simulink model "SDT505SimpleMotorModelPowerOutput220119"  (R2022b)
settings: Solver=VariableStepAuto  StartTime=0.0  StopTime=10.0  RelTol=1e-3
undefined symbols (not defined in the file or in its folder): m
libraries: simulink x4
settings Model: Creator=mjbou  LastModifiedBy=mjbou
settings SolverCC: AlgebraicLoopSolver=TrustRegion
settings DebuggingCC: UnconnectedInputMsg=warning  UnconnectedOutputMsg=warning  UnconnectedLineMsg=warning  SFMachineParentedDataDiag=warning
settings ModelReferenceCC: EnableRefExpFcnMdlSchedulingChecks=on

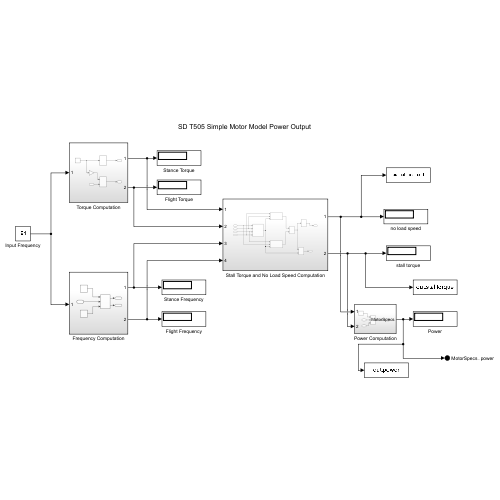
[thumbnail: Simulink's stored preview of the top-level diagram]
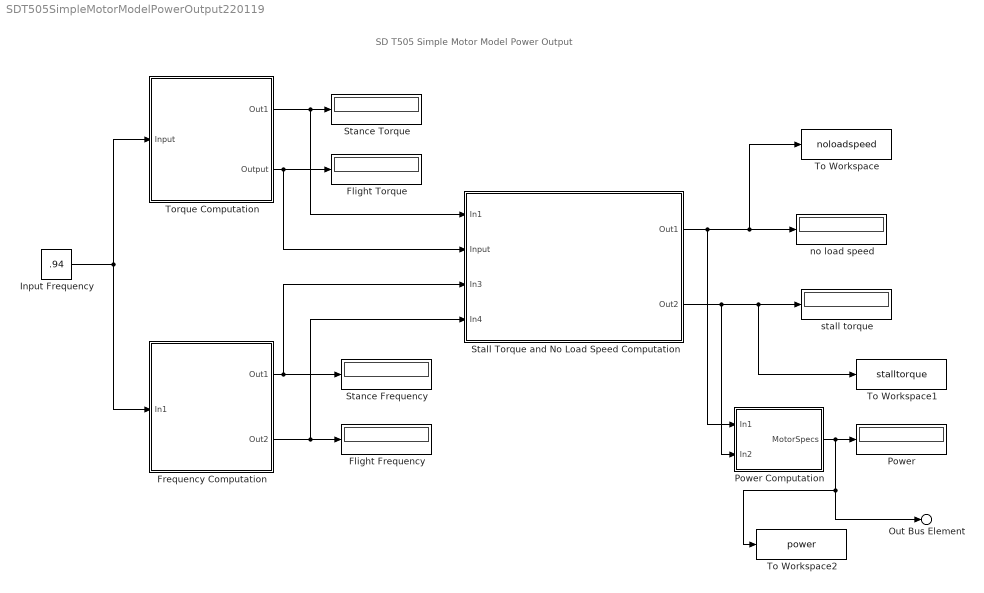
== system SDT505SimpleMotorModelPowerOutput220119 ==
  note: SD T505 Simple Motor Model Power Output
  Flight Frequency : Display
  Flight Torque : Display
  Frequency Computation : Subsystem
  Input Frequency : Constant  Value=.94
  Power : Display
  Power Computation : Subsystem
  Stall Torque and No Load Speed Computation : Subsystem
  Stance Frequency : Display
  Stance Torque : Display
  To Workspace : ToWorkspace  VariableName=noloadspeed  SaveFormat=Timeseries  SampleTime=-1
  To Workspace1 : ToWorkspace  VariableName=stalltorque  SaveFormat=Timeseries  SampleTime=-1
  To Workspace2 : ToWorkspace  VariableName=power  SaveFormat=Timeseries  SampleTime=-1
  Torque Computation : Subsystem
  no load speed : Display
  stall torque : Display
  Out Bus Element : Outport  PortName=MotorSpecs  Element=power
  wires:
  Frequency Computation/2(Out2) -> Stall Torque and No Load Speed Computation/4(In4), Flight Frequency/1
  Input Frequency/1 -> Torque Computation/1(Input), Frequency Computation/1(In1)
  Torque Computation/1(Out1) -> Stance Torque/1, Stall Torque and No Load Speed Computation/1(In1)
  Torque Computation/2(Output) -> Flight Torque/1, Stall Torque and No Load Speed Computation/2(Input)
  Stall Torque and No Load Speed Computation/1(Out1) -> Power Computation/1(In1), To Workspace/1, no load speed/1
  Stall Torque and No Load Speed Computation/2(Out2) -> Power Computation/2(In2), To Workspace1/1, stall torque/1
  Frequency Computation/1(Out1) -> Stance Frequency/1, Stall Torque and No Load Speed Computation/3(In3)
  Power Computation/1(MotorSpecs) -> To Workspace2/1, Out Bus Element/1, Power/1

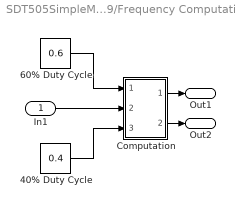
== system SDT505SimpleMotorModelPowerOutput220119/Frequency Computation ==
  In1 : Inport
  40% Duty Cycle : Constant  Value=0.4
  60% Duty Cycle : Constant  Value=0.6
  Computation : Subsystem
  Out1 : Outport
  Out2 : Outport  Port=2
  wires:
  60% Duty Cycle/1 -> Computation/1(In1)
  In1/1 -> Computation/2(In2)
  40% Duty Cycle/1 -> Computation/3(In3)
  Computation/1(Out1) -> Out1/1
  Computation/2(Out2) -> Out2/1

== system SDT505SimpleMotorModelPowerOutput220119/Power Computation ==
  In1 : Inport
  In2 : Inport  Port=2
  Constant : Constant  Value=0.25
  Product : Product  Inputs=3
  MotorSpecs : Outport
  wires:
  Constant/1 -> Product/1
  In2/1 -> Product/3
  In1/1 -> Product/2
  Product/1 -> MotorSpecs/1

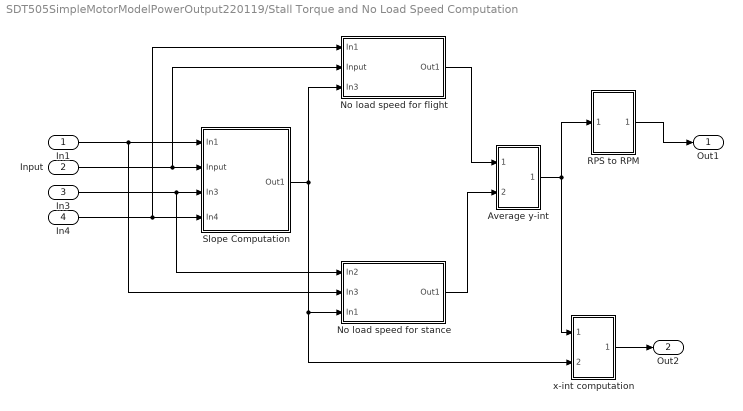
== system SDT505SimpleMotorModelPowerOutput220119/Stall Torque and No Load Speed Computation ==
  In1 : Inport
  Input : Inport  Port=2
  In3 : Inport  Port=3
  In4 : Inport  Port=4
  Average y-int : Subsystem
  No load speed for flight : Subsystem
  No load speed for stance : Subsystem
  RPS to RPM : Subsystem
  Slope Computation : Subsystem
  x-int computation : Subsystem
  Out1 : Outport
  Out2 : Outport  Port=2
  wires:
  No load speed for flight/1(Out1) -> Average y-int/1(In1)
  No load speed for stance/1(Out1) -> Average y-int/2(In2)
  Slope Computation/1(Out1) -> No load speed for flight/3(In3), x-int computation/2(In2), No load speed for stance/3(In1)
  x-int computation/1(Out1) -> Out2/1
  Average y-int/1(Out1) -> x-int computation/1(In1), RPS to RPM/1(In1)
  In3/1 -> No load speed for stance/1(In2), Slope Computation/3(In3)
  In1/1 -> No load speed for stance/2(In3), Slope Computation/1(In1)
  Input/1 -> No load speed for flight/2(Input), Slope Computation/2(Input)
  In4/1 -> No load speed for flight/1(In1), Slope Computation/4(In4)
  RPS to RPM/1(Out1) -> Out1/1

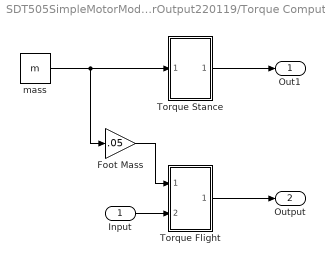
== system SDT505SimpleMotorModelPowerOutput220119/Torque Computation ==
  Input : Inport
  Foot Mass : Gain  Gain=.05
  Torque Flight : Subsystem
  Torque Stance : Subsystem
  mass : Constant  Value=m
  Out1 : Outport
  Output : Outport  Port=2
  wires:
  Torque Flight/1(Out2) -> Output/1
  Input/1 -> Torque Flight/2(Input)
  Torque Stance/1(Out1) -> Out1/1
  Foot Mass/1 -> Torque Flight/1(In1)
  mass/1 -> Foot Mass/1, Torque Stance/1(In1)

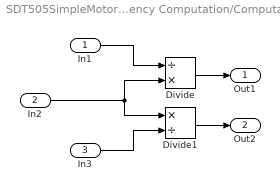
== system SDT505SimpleMotorModelPowerOutput220119/Frequency Computation/Computation ==
  In1 : Inport
  In2 : Inport  Port=2
  In3 : Inport  Port=3
  Divide : Product  Inputs=/*
  Divide1 : Product  Inputs=*/
  Out1 : Outport
  Out2 : Outport  Port=2
  wires:
  In2/1 -> Divide1/1, Divide/2
  Divide/1 -> Out1/1
  In3/1 -> Divide1/2
  In1/1 -> Divide/1
  Divide1/1 -> Out2/1

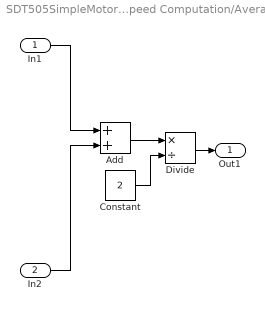
== system SDT505SimpleMotorModelPowerOutput220119/Stall Torque and No Load Speed Computation/Average y-int ==
  In1 : Inport
  In2 : Inport  Port=2
  Add : Sum
  Constant : Constant  Value=2
  Divide : Product  Inputs=*/
  Out1 : Outport
  wires:
  Divide/1 -> Out1/1
  Constant/1 -> Divide/2
  Add/1 -> Divide/1
  In1/1 -> Add/1
  In2/1 -> Add/2

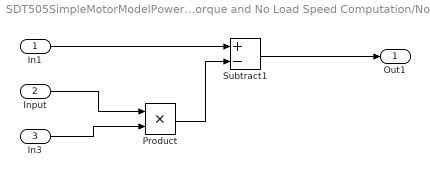
== system SDT505SimpleMotorModelPowerOutput220119/Stall Torque and No Load Speed Computation/No load speed for flight ==
  In1 : Inport
  Input : Inport  Port=2
  In3 : Inport  Port=3
  Product : Product
  Subtract1 : Sum  Inputs=+-
  Out1 : Outport
  wires:
  Input/1 -> Product/1
  In3/1 -> Product/2
  In1/1 -> Subtract1/1
  Product/1 -> Subtract1/2
  Subtract1/1 -> Out1/1

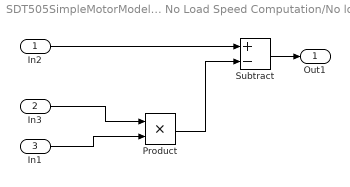
== system SDT505SimpleMotorModelPowerOutput220119/Stall Torque and No Load Speed Computation/No load speed for stance ==
  In2 : Inport
  In3 : Inport  Port=2
  In1 : Inport  Port=3
  Product : Product
  Subtract : Sum  Inputs=+-
  Out1 : Outport
  wires:
  Subtract/1 -> Out1/1
  Product/1 -> Subtract/2
  In3/1 -> Product/1
  In1/1 -> Product/2
  In2/1 -> Subtract/1

== system SDT505SimpleMotorModelPowerOutput220119/Stall Torque and No Load Speed Computation/RPS to RPM ==
  In1 : Inport
  Constant : Constant  Value=60
  Product : Product
  Out1 : Outport
  wires:
  In1/1 -> Product/2
  Product/1 -> Out1/1
  Constant/1 -> Product/1

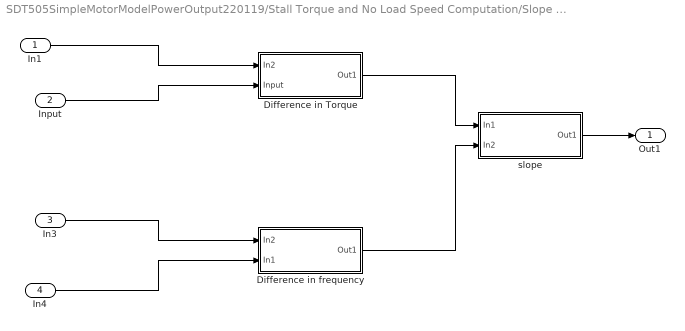
== system SDT505SimpleMotorModelPowerOutput220119/Stall Torque and No Load Speed Computation/Slope Computation ==
  In1 : Inport
  Input : Inport  Port=2
  In3 : Inport  Port=3
  In4 : Inport  Port=4
  Difference in Torque : Subsystem
  Difference in frequency : Subsystem
  slope : Subsystem
  Out1 : Outport
  wires:
  Difference in frequency/1(Out1) -> slope/2(In2)
  Difference in Torque/1(Out1) -> slope/1(In1)
  slope/1(Out1) -> Out1/1
  Input/1 -> Difference in Torque/2(Input)
  In4/1 -> Difference in frequency/2(In1)
  In1/1 -> Difference in Torque/1(In2)
  In3/1 -> Difference in frequency/1(In2)

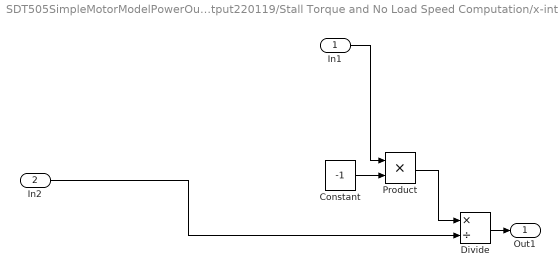
== system SDT505SimpleMotorModelPowerOutput220119/Stall Torque and No Load Speed Computation/x-int computation ==
  In1 : Inport
  In2 : Inport  Port=2
  Constant : Constant  Value=-1
  Divide : Product  Inputs=*/
  Product : Product
  Out1 : Outport
  wires:
  Constant/1 -> Product/2
  In1/1 -> Product/1
  Product/1 -> Divide/1
  In2/1 -> Divide/2
  Divide/1 -> Out1/1

== system SDT505SimpleMotorModelPowerOutput220119/Torque Computation/Torque Flight ==
  In1 : Inport
  Input : Inport  Port=2
  Angular Acceleration : Subsystem
  Computation : Subsystem
  Moment of Inertia : Subsystem
  Out2 : Outport
  wires:
  Moment of Inertia/1(Out1) -> Computation/1(In1)
  Angular Acceleration/1(Out1) -> Computation/2(In2)
  Computation/1(Out1) -> Out2/1
  Input/1 -> Angular Acceleration/1(Input)
  In1/1 -> Moment of Inertia/1(In1)

== system SDT505SimpleMotorModelPowerOutput220119/Torque Computation/Torque Stance ==
  In1 : Inport
  Computation : Subsystem
  Length : Subsystem
  Weight : Subsystem
  Out1 : Outport
  wires:
  Weight/1(Out1) -> Computation/1(In1)
  Length/1(Out1) -> Computation/2(In2)
  Computation/1(Out1) -> Out1/1
  In1/1 -> Weight/1(In1)

== system SDT505SimpleMotorModelPowerOutput220119/Stall Torque and No Load Speed Computation/Slope Computation/Difference in Torque ==
  In2 : Inport
  Input : Inport  Port=2
  Subtract1 : Sum  Inputs=+-
  Out1 : Outport
  wires:
  Subtract1/1 -> Out1/1
  Input/1 -> Subtract1/1
  In2/1 -> Subtract1/2

== system SDT505SimpleMotorModelPowerOutput220119/Stall Torque and No Load Speed Computation/Slope Computation/Difference in frequency ==
  In2 : Inport
  In1 : Inport  Port=2
  Subtract1 : Sum  Inputs=+-
  Out1 : Outport
  wires:
  Subtract1/1 -> Out1/1
  In1/1 -> Subtract1/1
  In2/1 -> Subtract1/2

== system SDT505SimpleMotorModelPowerOutput220119/Stall Torque and No Load Speed Computation/Slope Computation/slope ==
  In1 : Inport
  In2 : Inport  Port=2
  Divide : Product  Inputs=*/
  Out1 : Outport
  wires:
  In2/1 -> Divide/1
  In1/1 -> Divide/2
  Divide/1 -> Out1/1

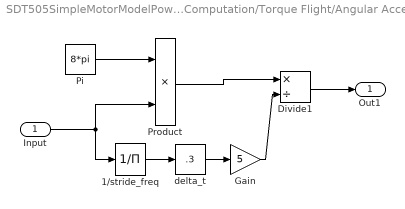
== system SDT505SimpleMotorModelPowerOutput220119/Torque Computation/Torque Flight/Angular Acceleration ==
  Input : Inport
  1/stride_freq : Product  Inputs=/
  Divide1 : Product  Inputs=*/
  Gain : Gain  Gain=5
  Pi : Constant  Value=8*pi  OutDataTypeStr=Inherit: Inherit via back propagation
  Product : Product
  delta_t : simulink/Math Operations/Slider Gain  gain=.3  low=0  high=2
  Out1 : Outport
  wires:
  Divide1/1 -> Out1/1
  Pi/1 -> Product/1
  delta_t/1 -> Gain/1
  1/stride_freq/1 -> delta_t/1
  Gain/1 -> Divide1/2
  Product/1 -> Divide1/1
  Input/1 -> Product/2, 1/stride_freq/1

== system SDT505SimpleMotorModelPowerOutput220119/Torque Computation/Torque Flight/Computation ==
  In1 : Inport
  In2 : Inport  Port=2
  Product1 : Product
  Torque stride : Display
  Out1 : Outport
  wires:
  Product1/1 -> Out1/1, Torque stride/1
  In2/1 -> Product1/2
  In1/1 -> Product1/1

== system SDT505SimpleMotorModelPowerOutput220119/Torque Computation/Torque Flight/Moment of Inertia ==
  In1 : Inport
  Constant1 : Constant
  L : simulink/Math Operations/Slider Gain  gain=0.2  low=0  high=2
  Product2 : Product
  Square : Math  Operator=square
  Out1 : Outport
  wires:
  Product2/1 -> Out1/1
  Square/1 -> Product2/1
  Constant1/1 -> L/1
  L/1 -> Square/1
  In1/1 -> Product2/2

== system SDT505SimpleMotorModelPowerOutput220119/Torque Computation/Torque Stance/Computation ==
  In1 : Inport
  In2 : Inport  Port=2
  Product3 : Product
  Torque stance : Display
  Out1 : Outport
  wires:
  Product3/1 -> Out1/1, Torque stance/1
  In1/1 -> Product3/1
  In2/1 -> Product3/2

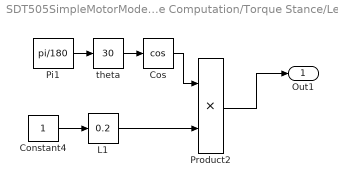
== system SDT505SimpleMotorModelPowerOutput220119/Torque Computation/Torque Stance/Length ==
  Constant4 : Constant
  Cos : Trigonometry  Operator=cos
  L1 : simulink/Math Operations/Slider Gain  gain=0.2  low=0  high=2
  Pi1 : Constant  Value=pi/180  OutDataTypeStr=Inherit: Inherit via back propagation
  Product2 : Product
  theta : simulink/Math Operations/Slider Gain  gain=30  low=0  high=360
  Out1 : Outport
  wires:
  Constant4/1 -> L1/1
  Product2/1 -> Out1/1
  Pi1/1 -> theta/1
  L1/1 -> Product2/2
  Cos/1 -> Product2/1
  theta/1 -> Cos/1

== system SDT505SimpleMotorModelPowerOutput220119/Torque Computation/Torque Stance/Weight ==
  In1 : Inport
  Gain : Gain  Gain=1.5
  Product1 : Product
  g1 : Constant  Value=9.81
  Out1 : Outport
  wires:
  g1/1 -> Product1/1
  Gain/1 -> Product1/2
  Product1/1 -> Out1/1
  In1/1 -> Gain/1
